simulink model "WholeSystemToPLC"  (R2021b)
settings: Solver=VariableStepAuto  StartTime=0.0  StopTime=10.0  RelTol=1e-3
undefined symbols (not defined in the file): A, a, beta, D_P, FL, k_EV, k_RV, m1, p_crackRV, V_pressure, xmax
libraries: slpidlib x2
settings Model: Creator=rrai-HIL  LastModifiedBy=rrai-HIL
settings ConfigComp: PLC_TargetIDE=codesys23  PLC_MultiTBSigbuilderTimeRange=off  PLC_InlineEnumCastFunction=off

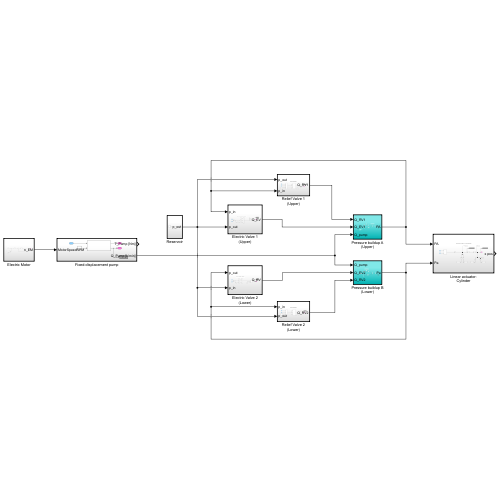
[thumbnail: Simulink's stored preview of the top-level diagram]
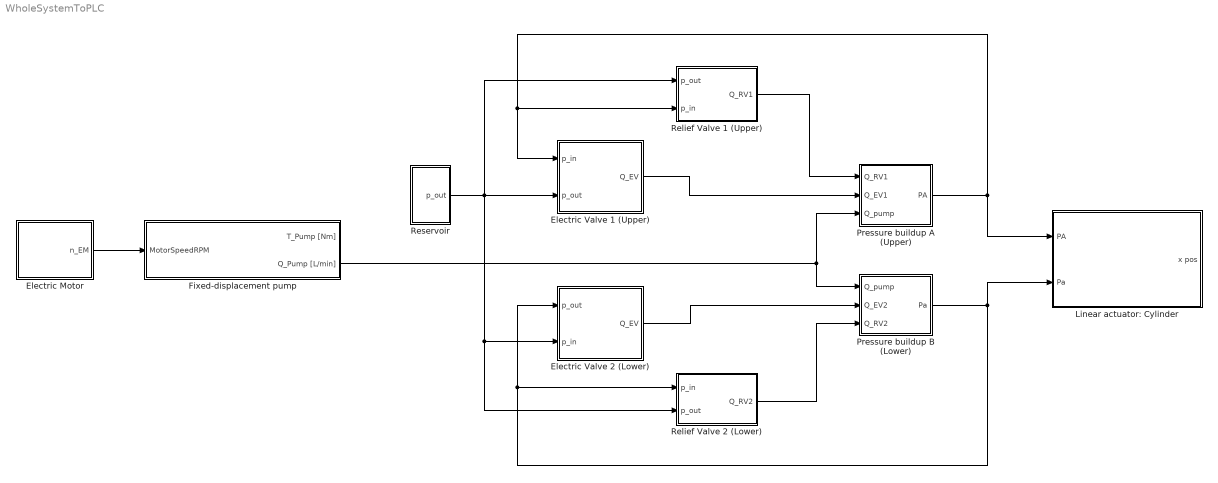
== system WholeSystemToPLC ==
  Electric Motor : Subsystem  TreatAsAtomicUnit=on
  Electric Valve 1 (Upper) : Subsystem  TreatAsAtomicUnit=on
  Electric Valve 2 (Lower) : Subsystem  TreatAsAtomicUnit=on
  Fixed-displacement pump : Subsystem  TreatAsAtomicUnit=on
  Linear actuator: Cylinder : Subsystem  TreatAsAtomicUnit=on
  Pressure buildup A (Upper) : Subsystem  TreatAsAtomicUnit=on
  Pressure buildup B (Lower) : Subsystem  TreatAsAtomicUnit=on
  Relief Valve 1 (Upper) : Subsystem  TreatAsAtomicUnit=on
  Relief Valve 2 (Lower) : Subsystem  TreatAsAtomicUnit=on
  Reservoir : Subsystem  TreatAsAtomicUnit=on
  wires:
  Reservoir/1(p_out) -> Electric Valve 1 (Upper)/2(p_out), Relief Valve 1 (Upper)/1(p_out), Electric Valve 2 (Lower)/2(p_in), Relief Valve 2 (Lower)/2(p_out)
  Electric Valve 2 (Lower)/1(Q_EV) -> Pressure buildup B (Lower)/2(Q_EV2)
  Relief Valve 1 (Upper)/1(Q_RV1) -> Pressure buildup A (Upper)/1(Q_RV1)
  Fixed-displacement pump/2(Q_Pump [L/min]) -> Pressure buildup A (Upper)/3(Q_pump), Pressure buildup B (Lower)/1(Q_pump)
  Relief Valve 2 (Lower)/1(Q_RV2) -> Pressure buildup B (Lower)/3(Q_RV2)
  Electric Valve 1 (Upper)/1(Q_EV) -> Pressure buildup A (Upper)/2(Q_EV1)
  Pressure buildup A (Upper)/1(PA) -> Electric Valve 1 (Upper)/1(p_in), Relief Valve 1 (Upper)/2(p_in), Linear actuator: Cylinder/1(PA)
  Pressure buildup B (Lower)/1(Pa) -> Electric Valve 2 (Lower)/1(p_out), Relief Valve 2 (Lower)/1(p_in), Linear actuator: Cylinder/2(Pa)
  Electric Motor/1(n_EM) -> Fixed-displacement pump/1(MotorSpeedRPM)

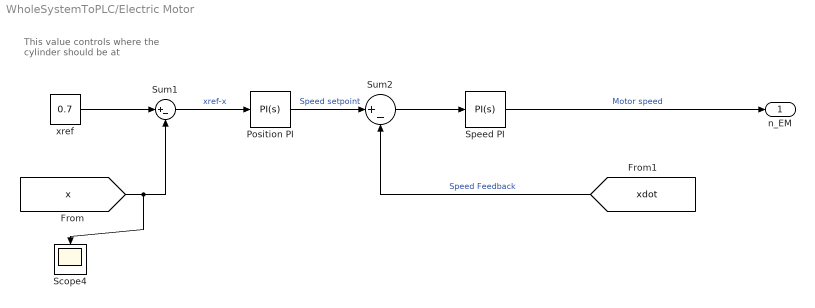
== system WholeSystemToPLC/Electric Motor ==
  note: This value controls
      | where the cylinder
      | should be at
  Position PI : slpidlib/PID Controller  Controller=PI  Form=Parallel  TimeDomain=Continuous-time  UseExternalTs=off  SampleTime=-1  IntegratorMethod=Forward Euler  FilterMethod=Forward Euler  ControllerParametersSource=internal  P=5  I=0.001  D=0  UseFilter=on  N=100  TunerSelectOption=Transfer Function Based (PID Tuner App)  InitialConditionSource=internal  InitialConditionForIntegrator=0  InitialConditionForFilter=0  DifferentiatorICPrevScaledInput=0  ExternalReset=none  TrackingMode=off  Kt=1  LimitOutput=on  SatLimitsSource=internal  UpperSaturationLimit=0.23  LowerSaturationLimit=-0.23  LinearizeAsGain=on  AntiWindupMode=none  Kb=1  POutMin=[]  POutMax=[]  IOutMin=[]  IOutMax=[]  DOutMin=[]  DOutMax=[]  NOutMin=[]  NOutMax=[]  SumOutMin=[]  SumOutMax=[]  SaturationOutMin=[]  SaturationOutMax=[]  PParamMin=[]  PParamMax=[]  IParamMin=[]  IParamMax=[]  DParamMin=[]  DParamMax=[]  NParamMin=[]  NParamMax=[]  KbParamMin=[]  KbParamMax=[]  KtParamMin=[]  KtParamMax=[]  KbOutMin=[]  KbOutMax=[]  KtOutMin=[]  KtOutMax=[]  IntegratorOutMin=[]  IntegratorOutMax=[]  FilterOutMin=[]  FilterOutMax=[]  SumI1OutMin=[]  SumI1OutMax=[]  SumI2OutMin=[]  SumI2OutMax=[]  SumI3OutMin=[]  SumI3OutMax=[]  SumI4OutMin=[]  SumI4OutMax=[]  SumDOutMin=[]  SumDOutMax=[]  DifferentiatorOutMin=[]  DifferentiatorOutMax=[]  FilterDiffOutCoefMin=[]  FilterDiffOutCoefMax=[]  ReciprocalOutMin=[]  ReciprocalOutMax=[]  SumDenOutMin=[]  SumDenOutMax=[]  SumNumOutMin=[]  SumNumOutMax=[]  DivideOutMin=[]  DivideOutMax=[]  UdiffTsProdOutMin=[]  UdiffTsProdOutMax=[]  NTsProdOutMin=[]  NTsProdOutMax=[]  UintegralTsProdOutMin=[]  UintegralTsProdOutMax=[]  UngainTsProdOutMin=[]  UngainTsProdOutMax=[]  IntegratorContinuousStateAttributes=''  IntegratorStateMustResolveToSignalObject=off  IntegratorRTWStateStorageClass=Auto  FilterContinuousStateAttributes=''  FilterStateMustResolveToSignalObject=off  FilterRTWStateStorageClass=Auto  ParallelPVariant=InternalParameters  IdealPVariant=Disabled  IVariant=InternalParameters  DVariant=Disabled  IntegratorVariant=Continuous  SatVariant=Enabled  AWVariant=Passthrough  PCopyVariant=Disabled  TRVariant=Disabled  FdbkBlocksVariant=Forward  IdealPFdbkVariant=Disabled  SatFdbkVariant=Disabled  DerivativeFilterVariant=Disabled  NVariant=Disabled  NCopyVariant=Disabled_SignalSpec  FilterICVariant=Disabled  IntegratorICVariant=InternalICs  ExternalResetVariant=Disabled  TRSumVariant=Passthrough  SumFdbkVariant=Disabled  SumVariant=Sum_PI  TsampFilterVariant=InternalTs  TsampNgainVariant=Passthrough  TsampIntegralVariant=Passthrough  ExternalSaturationOutDataTypeStr=Inherit: Same as second input
  Scope4 : Scope
  Speed PI : slpidlib/PID Controller  Controller=PI  Form=Parallel  TimeDomain=Continuous-time  UseExternalTs=off  SampleTime=-1  IntegratorMethod=Forward Euler  FilterMethod=Forward Euler  ControllerParametersSource=internal  P=2000  I=0.01  D=0  UseFilter=on  N=100  TunerSelectOption=Transfer Function Based (PID Tuner App)  InitialConditionSource=internal  InitialConditionForIntegrator=0  InitialConditionForFilter=0  DifferentiatorICPrevScaledInput=0  ExternalReset=none  TrackingMode=off  Kt=1  LimitOutput=off  SatLimitsSource=internal  UpperSaturationLimit=0.23  LowerSaturationLimit=-0.23  LinearizeAsGain=on  AntiWindupMode=none  Kb=1  POutMin=[]  POutMax=[]  IOutMin=[]  IOutMax=[]  DOutMin=[]  DOutMax=[]  NOutMin=[]  NOutMax=[]  SumOutMin=[]  SumOutMax=[]  SaturationOutMin=[]  SaturationOutMax=[]  PParamMin=[]  PParamMax=[]  IParamMin=[]  IParamMax=[]  DParamMin=[]  DParamMax=[]  NParamMin=[]  NParamMax=[]  KbParamMin=[]  KbParamMax=[]  KtParamMin=[]  KtParamMax=[]  KbOutMin=[]  KbOutMax=[]  KtOutMin=[]  KtOutMax=[]  IntegratorOutMin=[]  IntegratorOutMax=[]  FilterOutMin=[]  FilterOutMax=[]  SumI1OutMin=[]  SumI1OutMax=[]  SumI2OutMin=[]  SumI2OutMax=[]  SumI3OutMin=[]  SumI3OutMax=[]  SumI4OutMin=[]  SumI4OutMax=[]  SumDOutMin=[]  SumDOutMax=[]  DifferentiatorOutMin=[]  DifferentiatorOutMax=[]  FilterDiffOutCoefMin=[]  FilterDiffOutCoefMax=[]  ReciprocalOutMin=[]  ReciprocalOutMax=[]  SumDenOutMin=[]  SumDenOutMax=[]  SumNumOutMin=[]  SumNumOutMax=[]  DivideOutMin=[]  DivideOutMax=[]  UdiffTsProdOutMin=[]  UdiffTsProdOutMax=[]  NTsProdOutMin=[]  NTsProdOutMax=[]  UintegralTsProdOutMin=[]  UintegralTsProdOutMax=[]  UngainTsProdOutMin=[]  UngainTsProdOutMax=[]  IntegratorContinuousStateAttributes=''  IntegratorStateMustResolveToSignalObject=off  IntegratorRTWStateStorageClass=Auto  FilterContinuousStateAttributes=''  FilterStateMustResolveToSignalObject=off  FilterRTWStateStorageClass=Auto  ParallelPVariant=InternalParameters  IdealPVariant=Disabled  IVariant=InternalParameters  DVariant=Disabled  IntegratorVariant=Continuous  SatVariant=Disabled  AWVariant=Passthrough  PCopyVariant=Disabled  TRVariant=Disabled  FdbkBlocksVariant=Forward  IdealPFdbkVariant=Disabled  SatFdbkVariant=Disabled  DerivativeFilterVariant=Disabled  NVariant=Disabled  NCopyVariant=Disabled_SignalSpec  FilterICVariant=Disabled  IntegratorICVariant=InternalICs  ExternalResetVariant=Disabled  TRSumVariant=Passthrough  SumFdbkVariant=Disabled  SumVariant=Sum_PI  TsampFilterVariant=InternalTs  TsampNgainVariant=Passthrough  TsampIntegralVariant=Passthrough  ExternalSaturationOutDataTypeStr=Inherit: Same as second input
  Sum1 : Sum  Inputs=|+-
  Sum2 : Sum  Inputs=|+-
  xref : Constant  Value=0.7
  n_EM : Outport
  wires:
  Sum2/1 -> Speed PI/1
  xref/1 -> Sum1/1
  Position PI/1 -> Sum2/1  "Speed setpoint"
  Speed PI/1 -> n_EM/1  "Motor speed"
  Sum1/1 -> Position PI/1  "xref-x"
  [x] -> Sum1/2, Scope4/1
  [xdot] -> Sum2/2  "Speed Feedback"

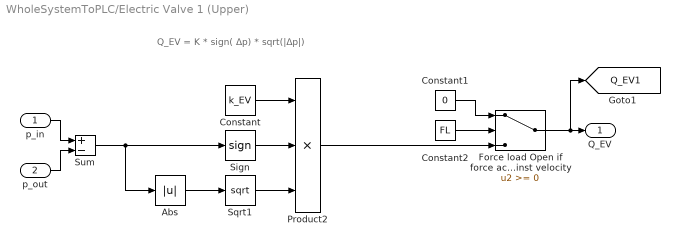
== system WholeSystemToPLC/Electric Valve 1 (Upper) ==
  note: Q_EV = K * sign( Δp) * sqrt(|Δp|)
  p_in : Inport
  p_out : Inport  Port=2
  Abs : Abs
  Constant : Constant  Value=k_EV
  Constant1 : Constant  Value=0
  Constant2 : Constant  Value=FL
  Force load Open if force acts against velocity : Switch
  Product2 : Product  Inputs=3
  Sign : Signum
  Sqrt1 : Sqrt  SaturateOnIntegerOverflow=on
  Sum : Sum  Inputs=+|-
  Q_EV : Outport
  tag scope: Q_EV1=global
  wires:
  Constant/1 -> Product2/1
  Sign/1 -> Product2/2
  Product2/1 -> Force load Open if force acts against velocity/3
  Sqrt1/1 -> Product2/3
  Abs/1 -> Sqrt1/1
  p_in/1 -> Sum/1
  Sum/1 -> Sign/1, Abs/1
  p_out/1 -> Sum/2
  Force load Open if force acts against velocity/1 -> [Q_EV1], Q_EV/1
  Constant2/1 -> Force load Open if force acts against velocity/2
  Constant1/1 -> Force load Open if force acts against velocity/1

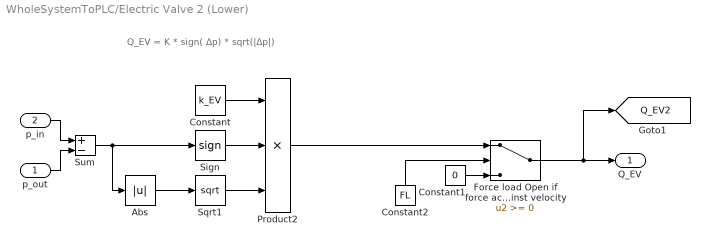
== system WholeSystemToPLC/Electric Valve 2 (Lower) ==
  note: Q_EV = K * sign( Δp) * sqrt(|Δp|)
  p_out : Inport
  p_in : Inport  Port=2
  Abs : Abs
  Constant : Constant  Value=k_EV
  Constant1 : Constant  Value=0
  Constant2 : Constant  Value=FL
  Force load Open if force acts against velocity : Switch
  Product2 : Product  Inputs=3
  Sign : Signum
  Sqrt1 : Sqrt  SaturateOnIntegerOverflow=on
  Sum : Sum  Inputs=+|-
  Q_EV : Outport
  tag scope: Q_EV2=global
  wires:
  Constant/1 -> Product2/1
  Sign/1 -> Product2/2
  Sqrt1/1 -> Product2/3
  Abs/1 -> Sqrt1/1
  p_in/1 -> Sum/1
  Sum/1 -> Abs/1, Sign/1
  p_out/1 -> Sum/2
  Constant1/1 -> Force load Open if force acts against velocity/3
  Product2/1 -> Force load Open if force acts against velocity/1
  Force load Open if force acts against velocity/1 -> [Q_EV2], Q_EV/1
  Constant2/1 -> Force load Open if force acts against velocity/2

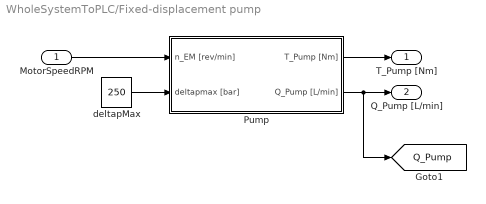
== system WholeSystemToPLC/Fixed-displacement pump ==
  MotorSpeedRPM : Inport
  Pump : Subsystem  TreatAsAtomicUnit=on
  deltapMax : Constant  Value=250
  T_Pump [Nm] : Outport
  Q_Pump [L/min] : Outport  Port=2
  tag scope: Q_Pump=global
  wires:
  Pump/1(T_Pump [Nm]) -> T_Pump [Nm]/1
  deltapMax/1 -> Pump/2(deltapmax [bar])
  MotorSpeedRPM/1 -> Pump/1(n_EM [rev/min])
  Pump/2(Q_Pump [L/min]) -> [Q_Pump], Q_Pump [L/min]/1

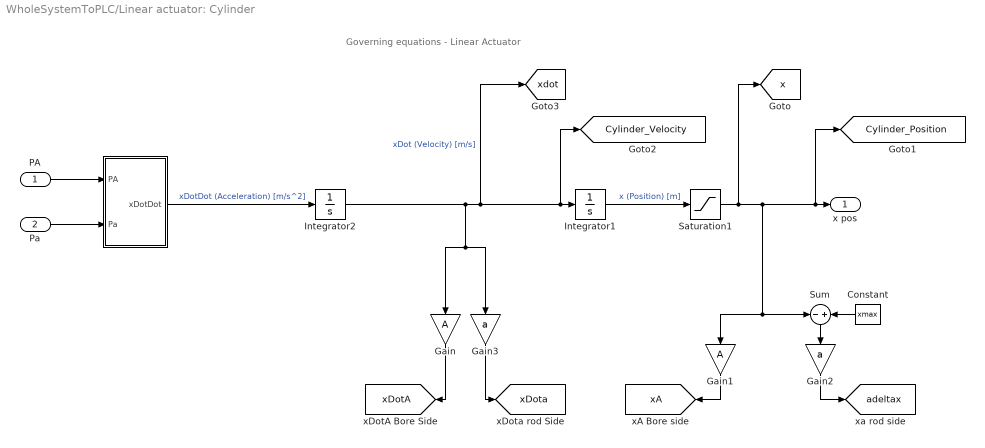
== system WholeSystemToPLC/Linear actuator: Cylinder ==
  note: Governing equations - Linear Actuator
  PA : Inport
  Pa : Inport  Port=2
  " " : Subsystem  TreatAsAtomicUnit=on
  Constant : Constant  Value=xmax
  Gain : Gain  Gain=A
  Gain1 : Gain  Gain=A
  Gain2 : Gain  Gain=a
  Gain3 : Gain  Gain=a
  Integrator1 : Integrator
  Integrator2 : Integrator
  Saturation1 : Saturate  UpperLimit=0.7  LowerLimit=-0.7
  Sum : Sum  Inputs=-|+
  x pos : Outport
  tag scope: Cylinder_Position=global, Cylinder_Velocity=global, adeltax=global, x=global, xA=global, xDotA=global, xDota=global, xdot=global
  wires:
  " "/1(xDotDot) -> Integrator2/1  "xDotDot (Acceleration) [m/s^2]"
  Integrator2/1 -> [xdot], Integrator1/1, [Cylinder_Velocity], Gain/1, Gain3/1  "xDot (Velocity) [m/s]"
  Integrator1/1 -> Saturation1/1  "x (Position) [m]"
  PA/1 -> " "/1(PA)
  Pa/1 -> " "/2(Pa)
  Gain/1 -> [xDotA]
  Gain1/1 -> [xA]
  Gain2/1 -> [adeltax]
  Gain3/1 -> [xDota]
  Sum/1 -> Gain2/1
  Constant/1 -> Sum/2
  Saturation1/1 -> [x], Sum/1, Gain1/1, [Cylinder_Position], x pos/1

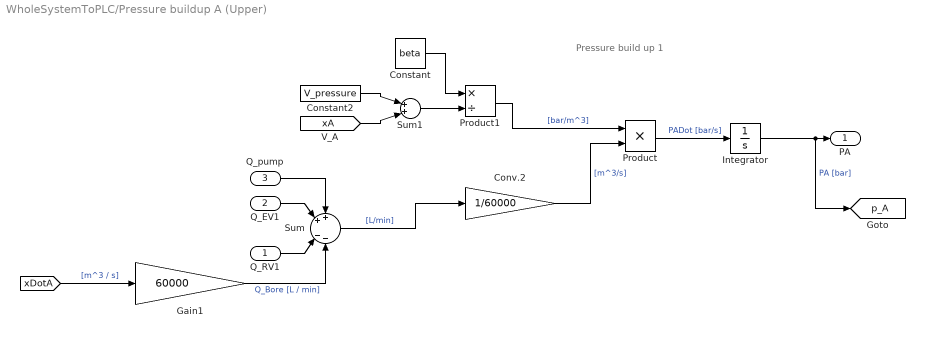
== system WholeSystemToPLC/Pressure buildup A (Upper) ==
  note: Pressure build up 1
  Q_RV1 : Inport
  Q_EV1 : Inport  Port=2
  Q_pump : Inport  Port=3
  Constant : Constant  Value=beta
  Constant2 : Constant  Value=V_pressure
  Conv.2 : Gain  Gain=1/60000
  Gain1 : Gain  Gain=60000
  Integrator : Integrator
  Product : Product
  Product1 : Product  Inputs=*/
  Sum : Sum  Inputs=++|--
  Sum1 : Sum  Inputs=|++|
  PA : Outport
  tag scope: p_A=global
  wires:
  Integrator/1 -> [p_A], PA/1  "PA [bar]"
  Q_pump/1 -> Sum/1
  Q_EV1/1 -> Sum/2
  Q_RV1/1 -> Sum/3
  Constant2/1 -> Sum1/1
  [xA] -> Sum1/2
  Product1/1 -> Product/1  "[bar/m^3]"
  Sum/1 -> Conv.2/1  "[L/min]"
  Product/1 -> Integrator/1  "PADot [bar/s]"
  [xDotA] -> Gain1/1  "[m^3 / s]"
  Gain1/1 -> Sum/4  "Q_Bore [L / min]"
  Conv.2/1 -> Product/2  "[m^3/s]"
  Constant/1 -> Product1/1
  Sum1/1 -> Product1/2

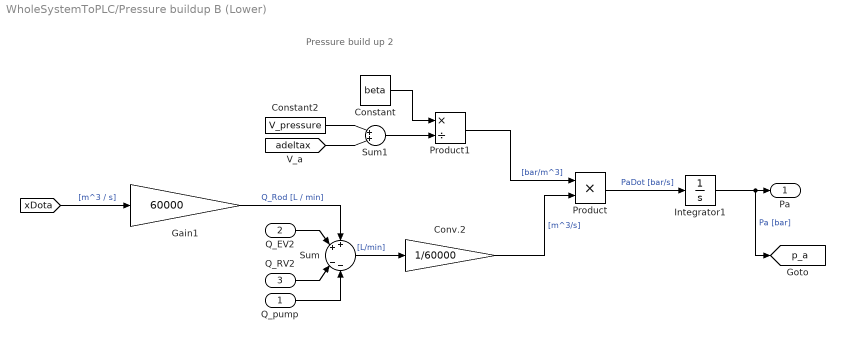
== system WholeSystemToPLC/Pressure buildup B (Lower) ==
  note: Pressure build up 2
  Q_pump : Inport
  Q_EV2 : Inport  Port=2
  Q_RV2 : Inport  Port=3
  Constant : Constant  Value=beta
  Constant2 : Constant  Value=V_pressure
  Conv.2 : Gain  Gain=1/60000
  Gain1 : Gain  Gain=60000
  Integrator1 : Integrator
  Product : Product
  Product1 : Product  Inputs=*/
  Sum : Sum  Inputs=++|--
  Sum1 : Sum  Inputs=|++|
  Pa : Outport
  tag scope: p_a=global
  wires:
  Product1/1 -> Product/1  "[bar/m^3]"
  Constant2/1 -> Sum1/1
  Q_EV2/1 -> Sum/2
  Sum/1 -> Conv.2/1  "[L/min]"
  [adeltax] -> Sum1/2
  Q_RV2/1 -> Sum/3
  Q_pump/1 -> Sum/4
  Product/1 -> Integrator1/1  "PaDot [bar/s]"
  Integrator1/1 -> [p_a], Pa/1  "Pa [bar]"
  [xDota] -> Gain1/1  "[m^3 / s]"
  Gain1/1 -> Sum/1  "Q_Rod [L / min]"
  Conv.2/1 -> Product/2  "[m^3/s]"
  Sum1/1 -> Product1/2
  Constant/1 -> Product1/1

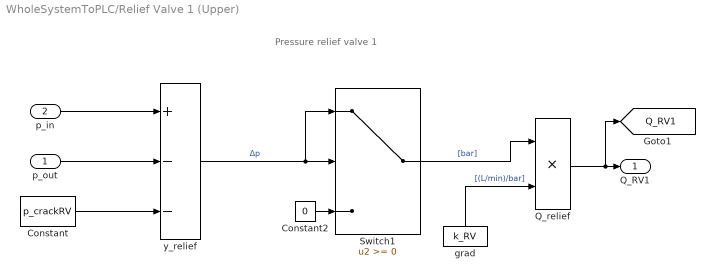
== system WholeSystemToPLC/Relief Valve 1 (Upper) ==
  note: Pressure relief valve 1
  p_out : Inport
  p_in : Inport  Port=2
  Constant : Constant  Value=p_crackRV
  Constant2 : Constant  Value=0
  Q_relief : Product  RndMeth=Zero
  Switch1 : Switch
  grad : Constant  Value=k_RV
  y_relief : Sum  Inputs=+--
  Q_RV1 : Outport  VectorParamsAs1DForOutWhenUnconnected=off
  tag scope: Q_RV1=global
  wires:
  y_relief/1 -> Switch1/1, Switch1/2  "Δp"
  Switch1/1 -> Q_relief/1  "[bar]"
  Q_relief/1 -> [Q_RV1], Q_RV1/1
  p_out/1 -> y_relief/2
  grad/1 -> Q_relief/2  "[(L/min)/bar]"
  Constant2/1 -> Switch1/3
  p_in/1 -> y_relief/1
  Constant/1 -> y_relief/3

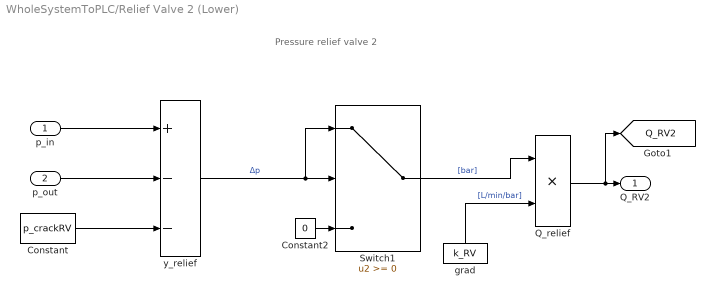
== system WholeSystemToPLC/Relief Valve 2 (Lower) ==
  note: Pressure relief valve 2
  p_in : Inport
  p_out : Inport  Port=2
  Constant : Constant  Value=p_crackRV
  Constant2 : Constant  Value=0
  Q_relief : Product  RndMeth=Zero
  Switch1 : Switch
  grad : Constant  Value=k_RV
  y_relief : Sum  Inputs=+--
  Q_RV2 : Outport  VectorParamsAs1DForOutWhenUnconnected=off
  tag scope: Q_RV2=global
  wires:
  Constant2/1 -> Switch1/3
  p_out/1 -> y_relief/2
  y_relief/1 -> Switch1/1, Switch1/2  "Δp"
  Switch1/1 -> Q_relief/1  "[bar]"
  p_in/1 -> y_relief/1
  grad/1 -> Q_relief/2  "[L/min/bar]"
  Constant/1 -> y_relief/3
  Q_relief/1 -> [Q_RV2], Q_RV2/1

== system WholeSystemToPLC/Reservoir ==
  Bar : Constant  Value=4
  p_out : Outport
  wires:
  Bar/1 -> p_out/1

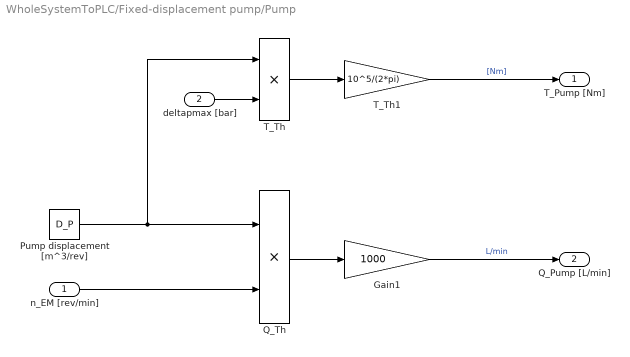
== system WholeSystemToPLC/Fixed-displacement pump/Pump ==
  n_EM [rev/min] : Inport
  deltapmax [bar] : Inport  Port=2
  Gain1 : Gain  Gain=1000
  Pump displacement [m^3/rev] : Constant  Value=D_P
  Q_Th : Product  RndMeth=Zero
  T_Th : Product  RndMeth=Zero
  T_Th1 : Gain  Gain=10^5/(2*pi)
  T_Pump [Nm] : Outport  VectorParamsAs1DForOutWhenUnconnected=off
  Q_Pump [L/min] : Outport  Port=2  VectorParamsAs1DForOutWhenUnconnected=off
  wires:
  Pump displacement [m^3/rev]/1 -> T_Th/1, Q_Th/1
  Q_Th/1 -> Gain1/1
  T_Th/1 -> T_Th1/1
  T_Th1/1 -> T_Pump [Nm]/1  "[Nm]"
  n_EM [rev/min]/1 -> Q_Th/2
  deltapmax [bar]/1 -> T_Th/2
  Gain1/1 -> Q_Pump [L/min]/1  "L/min"

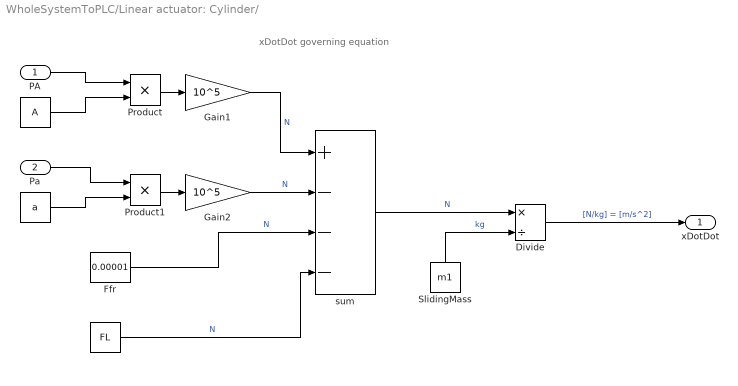
== system WholeSystemToPLC/Linear actuator: Cylinder/  ==
  note: xDotDot governing equation
  PA : Inport
  Pa : Inport  Port=2
  "   " : Constant  Value=A
  "    " : Constant  Value=a
  "      " : Constant  Value=FL
  "Divide " : Product  Inputs=*/
  Ffr : Constant  Value=0.00001
  Gain1 : Gain  Gain=10^5
  Gain2 : Gain  Gain=10^5
  Product : Product
  Product1 : Product
  SlidingMass : Constant  Value=m1
  sum : Sum  Inputs=+---
  xDotDot : Outport
  wires:
  Ffr/1 -> sum/3  "N"
  "   "/1 -> Product/2
  "    "/1 -> Product1/2
  Pa/1 -> Product1/1
  PA/1 -> Product/1
  SlidingMass/1 -> "Divide "/2  "kg"
  sum/1 -> "Divide "/1  "N"
  "      "/1 -> sum/4  "N"
  Product1/1 -> Gain2/1
  Gain2/1 -> sum/2  "N"
  Product/1 -> Gain1/1
  Gain1/1 -> sum/1  "N"
  "Divide "/1 -> xDotDot/1  "[N/kg] = [m/s^2]"
